simulink model "Traction_Control_main_code_Youla3"  (R2016a)
settings: Solver=VariableStepAuto  StartTime=0.0  StopTime=20  RelTol=1e-3
PreLoadFcn:
  | load('Traction_Control_parameter.mat')
values from neighbouring files (symbols this model uses):
  A = [0 -1; 4 -4]    [MAE298_HW5_Q2.m]    (also in MAE_272A_HW2_Q1a.m = 10; MAE_272A_HW2_Q4.m = [-2 -1 0; 1 0 0; 0 1 0]; MAE_272A_HW3_Q1a.m = 140; Traction_Control_Matlab_Youla.m = 70)
  alpha = 3600    [Traction_Control_parameter.mat]
  M = 50    [Traction_Control_parameter.mat]
  r = 0.26    [Traction_Control_parameter.mat]
  R = 2376    [Traction_Control_parameter.mat]
  T = minreal(1-S)    [MAE298_Final_Q2.m]    (also in MAE298_Final_Q22.m = 1-S; MAE298_Final_Q5.m = zpk(minreal(Y*Gp)); MAE_s72A_HW4_Q4.m = 1-S; MAE_s72A_HW4_Q4_5.m = 1-S)
  tau_tire = 0.1    [MAE_272A_HW3_Q1a.m]    (also in Traction_Control_Matlab_Youla.m; Traction_Control_Testing_main_3_1_17.m)
  TR = 4.6    [Traction_Control_parameter.mat]
  wn = 10.95    [MAE298_Final_Q5.m]    (also in MAE_272A_HW3_Q1a.m = 70; Traction_Control_Matlab_Youla.m = 70; Traction_Control_Testing_main_3_1_17.m = 1; Traction_Control_parameter.mat = 1)
  zeta = 0.707    [MAE298_Final_Q5.m]    (also in MAE_272A_HW3_Q1a.m = 1; Traction_Control_Matlab_Youla.m = 1; Traction_Control_Testing_main_3_1_17.m)
undefined symbols (not defined in the file or in its folder): sigbuilder_block
settings Model: Creator=Ping  LastModifiedBy=Ping

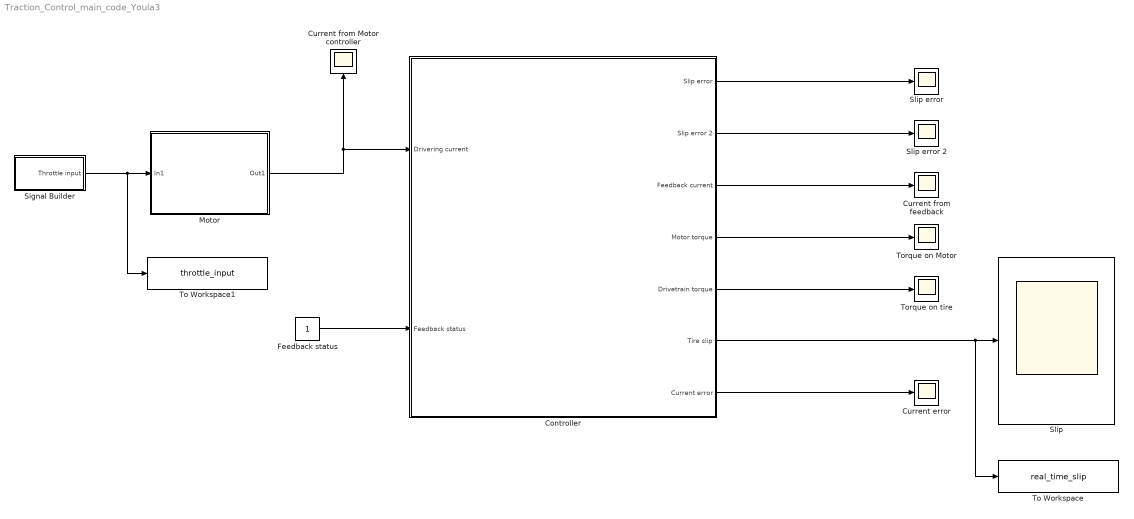
== system Traction_Control_main_code_Youla3 ==
  Controller : Subsystem
  Current error : Scope
  Current from Motor controller : Scope
  Current from feedback : Scope
  Feedback status : Constant
  Motor : Subsystem
  Signal Builder : Subsystem  Tag=STV Subsys  LoadFcn=sigbuilder_block('load');  StartFcn=sigbuilder_block('start');  StopFcn=sigbuilder_block('stop');  ClipboardFcn=sigbuilder_block('clipboard');  mask(Sigbuilder block){}
      mask help: Simulink:masks:SigbuilderBlock_MD
      mask init:
      | if ~strcmp(get_param(bdroot(gcbh),'SimulationStatus'),'stopped') tuvar = sigbuilder_block('maskInit'); end
      settings: CopyFcn=sigbuilder_block('copy');  DeleteFcn=sigbuilder_block('delete');  ModelCloseFcn=sigbuilder_block('modelClose');  PreSaveFcn=sigbuilder_block('preSave');  PauseFcn=sigbuilder_block('pause');  ContinueFcn=sigbuilder_block('continue');  NameChangeFcn=sigbuilder_block('namechange');  OpenFcn=sigbuilder_block('open',[118.5 71 550.5 362.5 ]);  CloseFcn=sigbuilder_block('close');
      mask Display: plot(0, 0, 100, 100,[2, 2, 32, 32, 2], [68, 8, 8, 68, 68],[32, 2], [38, 38], [32, 19, 2],[53, 60, 44], [32, 17, 17, 2],[16, 16, 31, 31]);txt = getActiveGroup(gcbh);text(2, 100, txt,'verticalAlignment', 'top');
  Slip : Scope
  Slip error : Scope
  Slip error 2 : Scope
  To Workspace : ToWorkspace  VariableName=real_time_slip  SaveFormat=Timeseries  SampleTime=-1
  To Workspace1 : ToWorkspace  VariableName=throttle_input  SaveFormat=Timeseries  SampleTime=-1
  Torque on Motor : Scope
  Torque on tire : Scope
  wires:
  Controller/1(Slip error) -> Slip error/1
  Controller/2(Slip error 2) -> Slip error 2/1
  Controller/3(Feedback current) -> Current from feedback/1
  Controller/4(Motor torque) -> Torque on Motor/1
  Controller/5(Drivetrain torque) -> Torque on tire/1
  Controller/6(Tire slip) -> To Workspace/1, Slip/1
  Motor/1(Out1) -> Current from Motor controller/1, Controller/1(Drivering current)
  Signal Builder/1(Throttle input) -> To Workspace1/1, Motor/1(In1)
  Controller/7(Current error) -> Current error/1
  Feedback status/1 -> Controller/2(Feedback status)

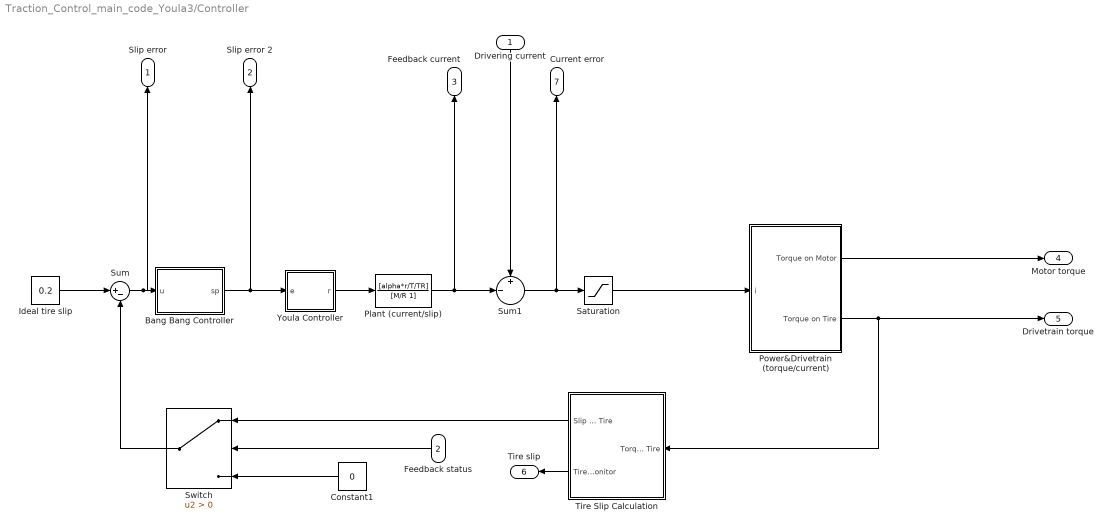
== system Traction_Control_main_code_Youla3/Controller ==
  Drivering current : Inport
  Feedback status : Inport  Port=2
  Bang Bang Controller : MATLAB Function  TreatAsAtomicUnit=on
  Constant1 : Constant  Value=0
  Ideal tire slip : Constant  Value=0.2
  Plant (current/slip) : TransferFcn  Numerator=[alpha*r/T/TR]  Denominator=[M/R 1]
  Power&Drivetrain (torque/current) : Subsystem
  Saturation : Saturate  UpperLimit=600  LowerLimit=0
  Sum : Sum  Inputs=|+-
  Sum1 : Sum  Inputs=+|-||
  Switch : Switch  Criteria=u2 > Threshold
  Tire Slip Calculation : Subsystem
  Youla Controller : Subsystem
  Slip error : Outport
  Slip error 2 : Outport  Port=2
  Feedback current : Outport  Port=3
  Motor torque : Outport  Port=4
  Drivetrain torque : Outport  Port=5
  Tire slip : Outport  Port=6
  Current error : Outport  Port=7
  wires:
  Plant (current/slip)/1 -> Sum1/2, Feedback current/1
  Sum1/1 -> Saturation/1, Current error/1
  Sum/1 -> Bang Bang Controller/1(u), Slip error/1
  Ideal tire slip/1 -> Sum/1
  Drivering current/1 -> Sum1/1
  Switch/1 -> Sum/2
  Constant1/1 -> Switch/3
  Feedback status/1 -> Switch/2
  Youla Controller/1(r) -> Plant (current/slip)/1
  Bang Bang Controller/1(sp) -> Youla Controller/1(e), Slip error 2/1
  Saturation/1 -> Power&Drivetrain (torque/current)/1(i)
  Power&Drivetrain (torque/current)/2(Torque on Tire) -> Tire Slip Calculation/1(Torque on Tire), Drivetrain torque/1
  Power&Drivetrain (torque/current)/1(Torque on Motor) -> Motor torque/1
  Tire Slip Calculation/1(Slip on Tire) -> Switch/1
  Tire Slip Calculation/2(Tire slip Monitor) -> Tire slip/1

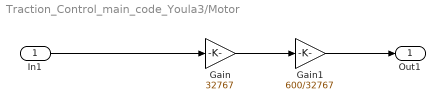
== system Traction_Control_main_code_Youla3/Motor ==
  In1 : Inport
  Gain : Gain  Gain=32767
  Gain1 : Gain  Gain=600/32767
  Out1 : Outport
  wires:
  Gain/1 -> Gain1/1
  In1/1 -> Gain/1
  Gain1/1 -> Out1/1

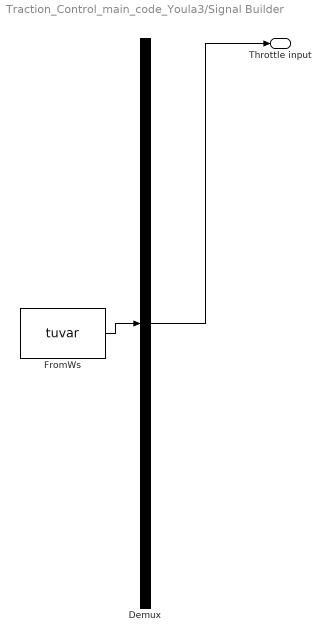
== system Traction_Control_main_code_Youla3/Signal Builder ==
  Demux : Demux  Tag=STV Demux  Outputs=1
  FromWs : FromWorkspace  Tag=STV FromWs  VariableName=tuvar  SampleTime=0
      SigBuilderData=|
      | common.afterFinalStr = 'Extrapolate'
      | common.sampleTime = 0
      | dataSet.timeRange = [0 20]
      | dataSet.name = 'Group 1'
      | sbobj.Groups.Name = 'Group 1'
      | sbobj.Groups.Signals.Name = 'Throttle input'
      | sbobj.Groups.Signals.XData = [0 4 4 12 12 20]
      | sbobj.Groups.Signals.YData = [0 0 1 1 0 0]
      | sbobj.Groups.TimeRange = [0 20]
  Throttle input : Outport  Tag=STV Outport
  wires:
  Demux/1 -> Throttle input/1
  FromWs/1 -> Demux/1

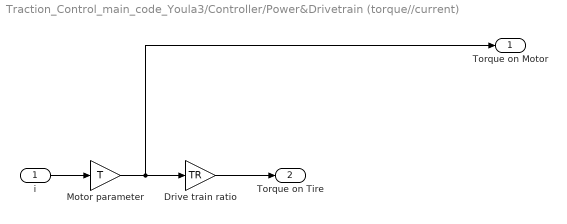
== system Traction_Control_main_code_Youla3/Controller/Power&Drivetrain (torque//current) ==
  i : Inport
  Drive train ratio : Gain  Gain=TR
  Motor parameter : Gain  Gain=T
  Torque on Motor : Outport
  Torque on Tire : Outport  Port=2
  wires:
  i/1 -> Motor parameter/1
  Motor parameter/1 -> Torque on Motor/1, Drive train ratio/1
  Drive train ratio/1 -> Torque on Tire/1

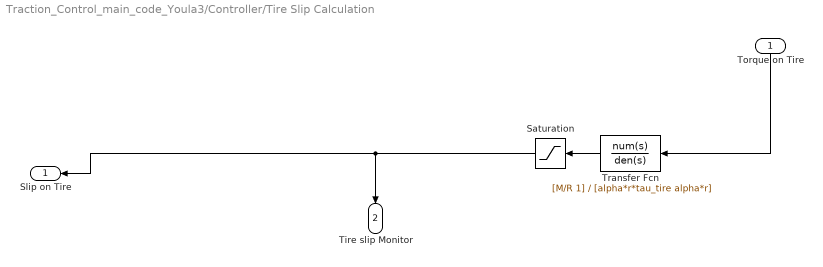
== system Traction_Control_main_code_Youla3/Controller/Tire Slip Calculation ==
  Torque on Tire : Inport
  Saturation : Saturate  UpperLimit=1  LowerLimit=0
  Transfer Fcn : TransferFcn  Numerator=[M/R 1]  Denominator=[alpha*r*tau_tire alpha*r]
  Slip on Tire : Outport
  Tire slip Monitor : Outport  Port=2
  wires:
  Torque on Tire/1 -> Transfer Fcn/1
  Transfer Fcn/1 -> Saturation/1
  Saturation/1 -> Tire slip Monitor/1, Slip on Tire/1

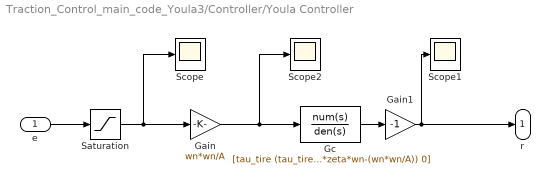
== system Traction_Control_main_code_Youla3/Controller/Youla Controller ==
  e : Inport
  Gain : Gain  Gain=wn*wn/A
      settings: AttributesFormatString=%<Gain>
  Gain1 : Gain  Gain=-1
  Gc : TransferFcn  Numerator=[tau_tire (tau_tire*A+1) A]  Denominator=[1 (2*zeta*wn-(wn*wn/A)) 0]
      settings: AttributesFormatString=|
      | num = %<Numerator>
      | den = %<Denominator>
  Saturation : Saturate  UpperLimit=0  LowerLimit=-1
  Scope : Scope
  Scope1 : Scope
  Scope2 : Scope
  r : Outport
  wires:
  e/1 -> Saturation/1
  Gc/1 -> Gain1/1
  Gain/1 -> Gc/1, Scope2/1
  Saturation/1 -> Scope/1, Gain/1
  Gain1/1 -> Scope1/1, r/1

== matlab function Traction_Control_main_code_Youla3/Controller/Bang Bang Controller ==
  data: u input; sp output
function sp = fcn(u)
%Only active while slip signal is negtive 
if u<0
    u_1 = u;
else 
    u_1 = 0;
end

sp = u_1;
